simulink model "step_ClosedLoopAngular"  (R2019a)
settings: Solver=VariableStepAuto  StartTime=0.0  StopTime=50.0  RelTol=1e-3
values from neighbouring files (symbols this model uses):
  den1 = [taum 1]    [classical.m]
  Kdin = (2*zetacin*wcin*Tm-1)/Km    [classical.m]
  Kpin = wcin^2*Tm/(Kdin*Km)    [classical.m]
  num1 = [Km1]    [classical.m]
settings Model: Creator=xde12  LastModifiedBy=xde12

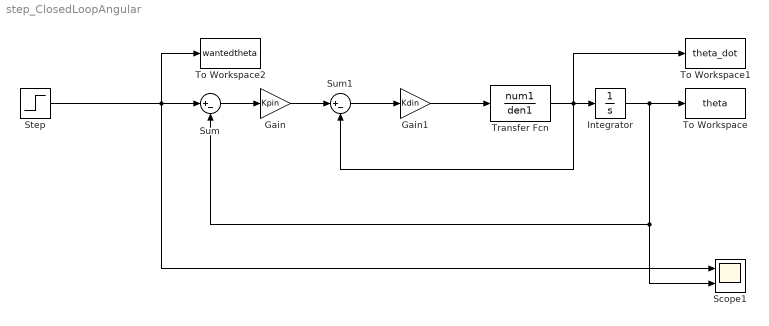
== system step_ClosedLoopAngular ==
  Gain : Gain  Gain=Kpin
  Gain1 : Gain  Gain=Kdin
  Integrator : Integrator
  Scope1 : Scope  NumInputPorts=2
  Step : Step  Time=0  After=30.0 / 180 *pi  SampleTime=0
  Sum : Sum  Inputs=|+-
  Sum1 : Sum  Inputs=|+-
  To Workspace : ToWorkspace  VariableName=theta  SampleTime=-1
  To Workspace1 : ToWorkspace  VariableName=theta_dot  SampleTime=-1
  To Workspace2 : ToWorkspace  VariableName=wantedtheta  SampleTime=-1
  Transfer Fcn : TransferFcn  Numerator=num1  Denominator=den1
  wires:
  Gain/1 -> Sum1/1
  Sum1/1 -> Gain1/1
  Gain1/1 -> Transfer Fcn/1
  Transfer Fcn/1 -> To Workspace1/1, Sum1/2, Integrator/1
  Integrator/1 -> To Workspace/1, Scope1/2, Sum/2
  Sum/1 -> Gain/1
  Step/1 -> To Workspace2/1, Scope1/1, Sum/1
